simulink model "automata_learning"  (R2022b)
settings: Solver=VariableStepAuto  StartTime=0.0  StopTime=10.0  RelTol=1e-3
settings Model: Creator=aaron  LastModifiedBy=aaron

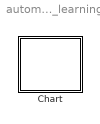
== system automata_learning ==
  Chart : Stateflow chart  TreatAsAtomicUnit=on

== stateflow chart automata_learning/Chart ==
